simulink model "LIPMobsv"  (R2018b)
settings: Solver=VariableStepAuto  StartTime=0.0  StopTime=10.0  RelTol=1e-3
values from neighbouring files (symbols this model uses):
  arm_radius = leg_radius    (= 0.01)    [Nao_paramter.m]
  foot_height = 0.02    [Nao_paramter.m]
  foot_length = 0.1    [Nao_paramter.m]
  foot_mass = 0.17184    [Nao_paramter.m]
  foot_width = 0.05    [Nao_paramter.m]
  ground_height = 0.0025    [Nao_paramter.m]
  ground_length = 5    [Nao_paramter.m]
  ground_width = 2    [Nao_paramter.m]
  hand_mass = 0.18533    [Nao_paramter.m]
  head_mass = 0.60533    [Nao_paramter.m]
  hip_mass = 0.14053    [Nao_paramter.m]
  hip_off_Y = 0.05    [Nao_paramter.m]
  hip_off_Z = 0.085    [Nao_paramter.m]
  leg_radius = 0.01    [Nao_paramter.m]
  lowerarm_length = 0.05595    [Nao_paramter.m]
  lowerarm_mass = 0.07761    [Nao_paramter.m]
  neck_length = 0.03    [Nao_paramter.m]
  neck_mass = 0.07842    [Nao_paramter.m]
  neck_off_Z = 0.1265    [Nao_paramter.m]
  shoulder_mass = 0.09304    [Nao_paramter.m]
  thigh_mass = 0.38968    [Nao_paramter.m]
  tibia_mass = 0.30142    [Nao_paramter.m]
  torso_height = foot_height + tibia_length + thigh_length + 0.5*hip_off_Z    (= 0.2654)    [Nao_paramter.m]
  torso_mass = 1.0496    [Nao_paramter.m]
  upperarm_length = 0.105    [Nao_paramter.m]
  upperarm_mass = 0.15777    [Nao_paramter.m]
undefined symbols (not defined in the file or in its folder): sigbuilder_block, X, Y, Z
libraries: sm_lib x166, nesl_utility x34, Contact_Forces_Lib x20
(part 6 of 6)

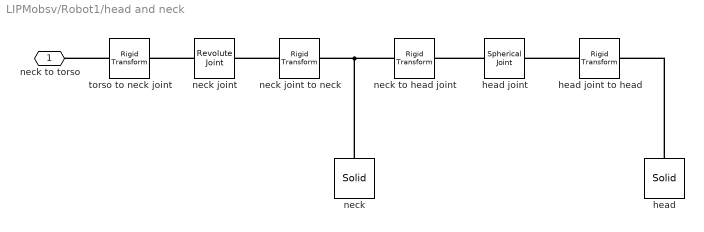
== system LIPMobsv/Robot1/head and neck ==
  head : sm_lib/Body Elements/Solid  InertiaType=CalculateFromGeometry  Mass=head_mass  MassUnits=kg  CenterOfMass=[0 0 0]  CenterOfMassUnits=m  MomentsOfInertia=[1 1 1]  MomentsOfInertiaUnits=kg*m^2  ProductsOfInertia=[1 1 1]  ProductsOfInertiaUnits=kg*m^2  BasedOnType=Mass  Density=1000  DensityUnits=kg/m^3  DoExposeReferenceFrame=on  SerializedFrames=<Frames/>  GraphicType=FromGeometry  MarkerShape=Sphere  MarkerSize=10  GraphicVisPropType=SimpleVisualProperties  GraphicDiffuseColor=[1.0 0.0 0.2]  GraphicSpecularColor=[0.5 0.5 0.5 1.0]  GraphicAmbientColor=[0.15 0.15 0.15 1.0]  GraphicEmissiveColor=[0.0 0.0 0.0 1.0]  GraphicShininess=75  GraphicOpacity=1.0  GeometryShape=Brick  RectangleSize=[1 1]  RectangleSizeUnits=m  BrickDimensions=[0.05 0.07 0.05]  BrickDimensionUnits=m  CylinderRadius=1  CylinderRadiusUnits=m  CylinderLength=1  CylinderLengthUnits=m  SphereRadius=1  SphereRadiusUnits=m  EllipsoidRadii=[1 1 1]  EllipsoidRadiiUnits=m  ExtrusionCrossSection=[1 1; -1 1; -1 -1; 1 -1]  ExtrusionCrossSectionUnits=m  ExtrusionLength=1  ExtrusionLengthUnits=m  PolygonNumSides=3  PolygonOuterRadius=1  PolygonOuterRadiusUnits=m  ExtGeomFileType=STEP  ExtGeomFileUnits=m  RevolutionCrossSection=[1 1; 1 -1; 2 -1; 2 1]  RevolutionCrossSectionUnits=m  RevolutionExtent=Full  RevolutionAngle=180  RevolutionAngleUnits=deg
  head joint : sm_lib/Joints/Spherical Joint  SenseConstraintForce=off  SenseConstraintForceX=off  SenseConstraintForceY=off  SenseConstraintForceZ=off  SenseConstraintTorque=off  SenseConstraintTorqueX=off  SenseConstraintTorqueY=off  SenseConstraintTorqueZ=off  SenseTotalForce=off  SenseTotalForceX=off  SenseTotalForceY=off  SenseTotalForceZ=off  SenseTotalTorque=off  SenseTotalTorqueX=off  SenseTotalTorqueY=off  SenseTotalTorqueZ=off  CompositeWrenchDir=FollowerOnBase  CompositeWrenchFrame=BaseFrame  DefPosRotationMethod=None  DefPosRotationAngleUnits=deg  DefPosRotationStandardAxis=+Z  DefPosRotationAngle=0.0  DefPosRotationArbitraryAxis=[0 0 1]  DefPosFollAlignAxisA=+X  DefPosBaseAlignAxisA=+Y  DefPosFollAlignAxisB=+Y  DefPosBaseAlignAxisB=+Z  DefPosRotationSequenceAxes=FollowerAxes  DefPosRotationSequence=XYX  DefPosRotationSequenceAngles=[0 0 0]  DefPosRotationSequenceAnglesUnits=deg  DefPosRotationMatrix=[1 0 0; 0 1 0; 0 0 1]  EqPosRotationMethod=None  EqPosRotationAngleUnits=deg  EqPosRotationStandardAxis=+Z  EqPosRotationAngle=0.0  EqPosRotationArbitraryAxis=[0 0 1]  EqPosFollAlignAxisA=+X  EqPosBaseAlignAxisA=+Y  EqPosFollAlignAxisB=+Y  EqPosBaseAlignAxisB=+Z  EqPosRotationSequenceAxes=FollowerAxes  EqPosRotationSequence=XYX  EqPosRotationSequenceAngles=[0 0 0]  EqPosRotationSequenceAnglesUnits=deg  EqPosRotationMatrix=[1 0 0; 0 1 0; 0 0 1]  SpringStiffness=0  SpringStiffnessUnits=N*m/deg  DampingCoefficient=0  DampingCoefficientUnits=N*m/(deg/s)  ActuateTorqueX=off  ActuateTorqueY=off  ActuateTorqueZ=off  ActuateTorque=off  TorqueActuationMode=NoTorque  MotionActuationMode=ComputedMotion  ActuationFrame=BaseFrame  SensePosition=off  SenseVelocityX=off  SenseVelocityY=off  SenseVelocityZ=off  SenseVelocity=off  SenseAccelerationX=off  SenseAccelerationY=off  SenseAccelerationZ=off  SenseAcceleration=off  SenseTorqueX=off  SenseTorqueY=off  SenseTorqueZ=off  SenseTorqueForce=off  SensingFrame=BaseFrame  PositionTargetRotationMethod=StandardAxis  PositionTargetRotationAngleUnits=deg  PositionTargetRotationStandardAxis=+Y  PositionTargetRotationAngle=5  PositionTargetRotationArbitraryAxis=[0 0 1]  PositionTargetFollAlignAxisA=+X  PositionTargetBaseAlignAxisA=+Y  PositionTargetFollAlignAxisB=+Y  PositionTargetBaseAlignAxisB=+Z  PositionTargetRotationSequenceAxes=FollowerAxes  PositionTargetRotationSequence=XYX  PositionTargetRotationSequenceAngles=[0 0 0]  PositionTargetRotationSequenceAnglesUnits=deg  PositionTargetRotationMatrix=[1 0 0; 0 1 0; 0 0 1]  PositionTargetSpecify=off  PositionTargetPriority=High  VelocityTargetValue=[0 0 0]  VelocityTargetValueUnits=deg/s  VelocityTargetSpecify=off  VelocityTargetPriority=High  VelocityTargetInFollowerFrame=on
  head joint to head : sm_lib/Frames and Transforms/Rigid Transform  TranslationMethod=StandardAxis  TranslationStandardOffset=0.025  TranslationLengthUnit=m  TranslationStandardAxis=+Z  TranslationCartesianOffset=[0 0 0]  TranslationROffset=0  TranslationROffsetUnits=m  TranslationZOffset=0  TranslationZOffsetUnits=m  TranslationThetaOffset=0  TranslationThetaOffsetUnits=deg  RotationMethod=None  RotationAngleUnits=deg  RotationStandardAxis=+Z  RotationAngle=0.0  RotationArbitraryAxis=[0 0 1]  FollAlignAxisA=+X  BaseAlignAxisA=+Y  FollAlignAxisB=+Y  BaseAlignAxisB=+Z  RotationSequenceAxes=FollowerAxes  RotationSequence=XYX  RotationSequenceAngles=[0 0 0]  RotationSequenceAnglesUnits=deg  RotationMatrix=[1 0 0; 0 1 0; 0 0 1]
  neck : sm_lib/Body Elements/Solid  InertiaType=CalculateFromGeometry  Mass=neck_mass  MassUnits=kg  CenterOfMass=[0 0 0]  CenterOfMassUnits=m  MomentsOfInertia=[1 1 1]  MomentsOfInertiaUnits=kg*m^2  ProductsOfInertia=[1 1 1]  ProductsOfInertiaUnits=kg*m^2  BasedOnType=Mass  Density=1000  DensityUnits=kg/m^3  DoExposeReferenceFrame=on  SerializedFrames=<Frames/>  GraphicType=FromGeometry  MarkerShape=Sphere  MarkerSize=10  GraphicVisPropType=SimpleVisualProperties  GraphicDiffuseColor=[0.5 0.5 0.5]  GraphicSpecularColor=[0.5 0.5 0.5 1.0]  GraphicAmbientColor=[0.15 0.15 0.15 1.0]  GraphicEmissiveColor=[0.0 0.0 0.0 1.0]  GraphicShininess=75  GraphicOpacity=1.0  GeometryShape=Cylinder  RectangleSize=[1 1]  RectangleSizeUnits=m  BrickDimensions=[1 1 1]  BrickDimensionUnits=m  CylinderRadius=neck_radius  CylinderRadiusUnits=m  CylinderLength=neck_length  CylinderLengthUnits=m  SphereRadius=1  SphereRadiusUnits=m  EllipsoidRadii=[1 1 1]  EllipsoidRadiiUnits=m  ExtrusionCrossSection=[1 1; -1 1; -1 -1; 1 -1]  ExtrusionCrossSectionUnits=m  ExtrusionLength=1  ExtrusionLengthUnits=m  PolygonNumSides=3  PolygonOuterRadius=1  PolygonOuterRadiusUnits=m  ExtGeomFileType=STEP  ExtGeomFileUnits=m  RevolutionCrossSection=[1 1; 1 -1; 2 -1; 2 1]  RevolutionCrossSectionUnits=m  RevolutionExtent=Full  RevolutionAngle=180  RevolutionAngleUnits=deg
  neck joint : sm_lib/Joints/Revolute Joint  SenseConstraintForce=off  SenseConstraintForceX=off  SenseConstraintForceY=off  SenseConstraintForceZ=off  SenseConstraintTorque=off  SenseConstraintTorqueX=off  SenseConstraintTorqueY=off  SenseConstraintTorqueZ=off  SenseTotalForce=off  SenseTotalForceX=off  SenseTotalForceY=off  SenseTotalForceZ=off  SenseTotalTorque=off  SenseTotalTorqueX=off  SenseTotalTorqueY=off  SenseTotalTorqueZ=off  CompositeWrenchDir=FollowerOnBase  CompositeWrenchFrame=BaseFrame  EquilibriumPosition=0  EquilibriumPositionUnits=deg  SpringStiffness=0  SpringStiffnessUnits=N*m/deg  DampingCoefficient=0  DampingCoefficientUnits=N*m/(deg/s)  TorqueActuationMode=NoTorque  MotionActuationMode=ComputedMotion  SensePosition=off  SenseVelocity=off  SenseAcceleration=off  SenseTorqueForce=off  PositionTargetSpecify=off  PositionTargetPriority=High  PositionTargetValue=0  PositionTargetValueUnits=deg  VelocityTargetSpecify=off  VelocityTargetPriority=High  VelocityTargetValue=0  VelocityTargetValueUnits=deg/s
  neck joint to neck : sm_lib/Frames and Transforms/Rigid Transform  TranslationMethod=None  TranslationStandardOffset=0  TranslationLengthUnit=m  TranslationStandardAxis=+Z  TranslationCartesianOffset=[0 0 0]  TranslationROffset=0  TranslationROffsetUnits=m  TranslationZOffset=0  TranslationZOffsetUnits=m  TranslationThetaOffset=0  TranslationThetaOffsetUnits=deg  RotationMethod=None  RotationAngleUnits=deg  RotationStandardAxis=+Z  RotationAngle=0.0  RotationArbitraryAxis=[0 0 1]  FollAlignAxisA=+X  BaseAlignAxisA=+Y  FollAlignAxisB=+Y  BaseAlignAxisB=+Z  RotationSequenceAxes=FollowerAxes  RotationSequence=XYX  RotationSequenceAngles=[0 0 0]  RotationSequenceAnglesUnits=deg  RotationMatrix=[1 0 0; 0 1 0; 0 0 1]
  neck to head joint : sm_lib/Frames and Transforms/Rigid Transform  TranslationMethod=StandardAxis  TranslationStandardOffset=neck_length/2  TranslationLengthUnit=m  TranslationStandardAxis=+Z  TranslationCartesianOffset=[0 0 0]  TranslationROffset=0  TranslationROffsetUnits=m  TranslationZOffset=0  TranslationZOffsetUnits=m  TranslationThetaOffset=0  TranslationThetaOffsetUnits=deg  RotationMethod=None  RotationAngleUnits=deg  RotationStandardAxis=+Z  RotationAngle=0.0  RotationArbitraryAxis=[0 0 1]  FollAlignAxisA=+X  BaseAlignAxisA=+Y  FollAlignAxisB=+Y  BaseAlignAxisB=+Z  RotationSequenceAxes=FollowerAxes  RotationSequence=XYX  RotationSequenceAngles=[0 0 0]  RotationSequenceAnglesUnits=deg  RotationMatrix=[1 0 0; 0 1 0; 0 0 1]
  torso to neck joint : sm_lib/Frames and Transforms/Rigid Transform  TranslationMethod=StandardAxis  TranslationStandardOffset=(hip_off_Z+neck_off_Z)/2  TranslationLengthUnit=m  TranslationStandardAxis=+Z  TranslationCartesianOffset=[0 0 0]  TranslationROffset=0  TranslationROffsetUnits=m  TranslationZOffset=0  TranslationZOffsetUnits=m  TranslationThetaOffset=0  TranslationThetaOffsetUnits=deg  RotationMethod=None  RotationAngleUnits=deg  RotationStandardAxis=+Z  RotationAngle=0.0  RotationArbitraryAxis=[0 0 1]  FollAlignAxisA=+X  BaseAlignAxisA=+Y  FollAlignAxisB=+Y  BaseAlignAxisB=+Z  RotationSequenceAxes=FollowerAxes  RotationSequence=XYX  RotationSequenceAngles=[0 0 0]  RotationSequenceAnglesUnits=deg  RotationMatrix=[1 0 0; 0 1 0; 0 0 1]
  neck to torso : PMIOPort  Side=Left
  connections:
  torso to neck joint/LConn1 -- neck to torso/RConn1
  neck joint/LConn1 -- torso to neck joint/RConn1
  neck joint to neck/LConn1 -- neck joint/RConn1
  neck/RConn1 -- neck to head joint/LConn1 -- neck joint to neck/RConn1
  head joint/LConn1 -- neck to head joint/RConn1
  head/RConn1 -- head joint to head/RConn1
  head joint to head/LConn1 -- head joint/RConn1

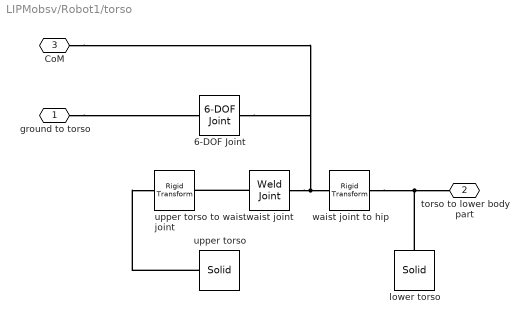
== system LIPMobsv/Robot1/torso ==
  " waist joint" : sm_lib/Joints/Weld Joint  SenseConstraintForce=off  SenseConstraintForceX=off  SenseConstraintForceY=off  SenseConstraintForceZ=off  SenseConstraintTorque=off  SenseConstraintTorqueX=off  SenseConstraintTorqueY=off  SenseConstraintTorqueZ=off  SenseTotalForce=off  SenseTotalForceX=off  SenseTotalForceY=off  SenseTotalForceZ=off  SenseTotalTorque=off  SenseTotalTorqueX=off  SenseTotalTorqueY=off  SenseTotalTorqueZ=off  CompositeWrenchDir=FollowerOnBase  CompositeWrenchFrame=BaseFrame
  6-DOF Joint : sm_lib/Joints/6-DOF Joint  SenseConstraintForce=off  SenseConstraintForceX=off  SenseConstraintForceY=off  SenseConstraintForceZ=off  SenseConstraintTorque=off  SenseConstraintTorqueX=off  SenseConstraintTorqueY=off  SenseConstraintTorqueZ=off  SenseTotalForce=off  SenseTotalForceX=off  SenseTotalForceY=off  SenseTotalForceZ=off  SenseTotalTorque=off  SenseTotalTorqueX=off  SenseTotalTorqueY=off  SenseTotalTorqueZ=off  CompositeWrenchDir=FollowerOnBase  CompositeWrenchFrame=BaseFrame  PxEquilibriumPosition=0  PxEquilibriumPositionUnits=m  PxSpringStiffness=1000  PxSpringStiffnessUnits=N/m  PxDampingCoefficient=800  PxDampingCoefficientUnits=N/(m/s)  PxTorqueActuationMode=NoTorque  PxMotionActuationMode=ComputedMotion  PxSensePosition=off  PxSenseVelocity=off  PxSenseAcceleration=off  PxSenseTorqueForce=off  PxPositionTargetSpecify=on  PxPositionTargetPriority=High  PxPositionTargetValue=0  PxPositionTargetValueUnits=m  PxVelocityTargetSpecify=off  PxVelocityTargetPriority=High  PxVelocityTargetValue=0  PxVelocityTargetValueUnits=m/s  PyEquilibriumPosition=0  PyEquilibriumPositionUnits=m  PySpringStiffness=1000  PySpringStiffnessUnits=N/m  PyDampingCoefficient=800  PyDampingCoefficientUnits=N/(m/s)  PyTorqueActuationMode=NoTorque  PyMotionActuationMode=ComputedMotion  PySensePosition=off  PySenseVelocity=off  PySenseAcceleration=off  PySenseTorqueForce=off  PyPositionTargetSpecify=on  PyPositionTargetPriority=High  PyPositionTargetValue=0  PyPositionTargetValueUnits=m  PyVelocityTargetSpecify=off  PyVelocityTargetPriority=High  PyVelocityTargetValue=0  PyVelocityTargetValueUnits=m/s  PzEquilibriumPosition=0  PzEquilibriumPositionUnits=m  PzSpringStiffness=1000  PzSpringStiffnessUnits=N/m  PzDampingCoefficient=800  PzDampingCoefficientUnits=N/(m/s)  PzTorqueActuationMode=NoTorque  PzMotionActuationMode=ComputedMotion  PzSensePosition=off  PzSenseVelocity=off  PzSenseAcceleration=off  PzSenseTorqueForce=off  PzPositionTargetSpecify=on  PzPositionTargetPriority=High  PzPositionTargetValue=torso_height+0.001  PzPositionTargetValueUnits=m  PzVelocityTargetSpecify=off  PzVelocityTargetPriority=High  PzVelocityTargetValue=0  PzVelocityTargetValueUnits=m/s  SphDefPosRotationMethod=None  SphDefPosRotationAngleUnits=deg  SphDefPosRotationStandardAxis=+Z  SphDefPosRotationAngle=0.0  SphDefPosRotationArbitraryAxis=[0 0 1]  SphDefPosFollAlignAxisA=+X  SphDefPosBaseAlignAxisA=+Y  SphDefPosFollAlignAxisB=+Y  SphDefPosBaseAlignAxisB=+Z  SphDefPosRotationSequenceAxes=FollowerAxes  SphDefPosRotationSequence=XYX  SphDefPosRotationSequenceAngles=[0 0 0]  SphDefPosRotationSequenceAnglesUnits=deg  SphDefPosRotationMatrix=[1 0 0; 0 1 0; 0 0 1]  SphEqPosRotationMethod=None  SphEqPosRotationAngleUnits=deg  SphEqPosRotationStandardAxis=+Z  SphEqPosRotationAngle=0.0  SphEqPosRotationArbitraryAxis=[0 0 1]  SphEqPosFollAlignAxisA=+X  SphEqPosBaseAlignAxisA=+Y  SphEqPosFollAlignAxisB=+Y  SphEqPosBaseAlignAxisB=+Z  SphEqPosRotationSequenceAxes=FollowerAxes  SphEqPosRotationSequence=XYX  SphEqPosRotationSequenceAngles=[0 0 0]  SphEqPosRotationSequenceAnglesUnits=deg  SphEqPosRotationMatrix=[1 0 0; 0 1 0; 0 0 1]  SphSpringStiffness=1000  SphSpringStiffnessUnits=N*m/deg  SphDampingCoefficient=1000  SphDampingCoefficientUnits=N*m/(rad/s)  SphActuateTorqueX=off  SphActuateTorqueY=off  SphActuateTorqueZ=off  SphActuateTorque=off  SphTorqueActuationMode=NoTorque  SphMotionActuationMode=ComputedMotion  SphActuationFrame=BaseFrame  SphSensePosition=off  SphSenseVelocityX=off  SphSenseVelocityY=off  SphSenseVelocityZ=off  SphSenseVelocity=off  SphSenseAccelerationX=off  SphSenseAccelerationY=off  SphSenseAccelerationZ=off  SphSenseAcceleration=off  SphSenseTorqueX=off  SphSenseTorqueY=off  SphSenseTorqueZ=off  SphSenseTorqueForce=off  SphSensingFrame=BaseFrame  SphPositionTargetRotationMethod=None  SphPositionTargetRotationAngleUnits=deg  SphPositionTargetRotationStandardAxis=+Z  SphPositionTargetRotationAngle=0.0  SphPositionTargetRotationArbitraryAxis=[0 0 1]  SphPositionTargetFollAlignAxisA=+X  SphPositionTargetBaseAlignAxisA=+Y  SphPositionTargetFollAlignAxisB=+Y  SphPositionTargetBaseAlignAxisB=+Z  SphPositionTargetRotationSequenceAxes=FollowerAxes  SphPositionTargetRotationSequence=XYX  SphPositionTargetRotationSequenceAngles=[0 0 0]  SphPositionTargetRotationSequenceAnglesUnits=deg  SphPositionTargetRotationMatrix=eye(3)  SphPositionTargetSpecify=off  SphPositionTargetPriority=High  SphVelocityTargetValue=[0 0 0]  SphVelocityTargetValueUnits=deg/s  SphVelocityTargetSpecify=off  SphVelocityTargetPriority=High  SphVelocityTargetInFollowerFrame=on
  lower torso : sm_lib/Body Elements/Solid  InertiaType=CalculateFromGeometry  Mass=hip_mass  MassUnits=kg  CenterOfMass=[0 0 0]  CenterOfMassUnits=m  MomentsOfInertia=[1 1 1]  MomentsOfInertiaUnits=kg*m^2  ProductsOfInertia=[1 1 1]  ProductsOfInertiaUnits=kg*m^2  BasedOnType=Mass  Density=1000  DensityUnits=kg/m^3  DoExposeReferenceFrame=on  SerializedFrames=<Frames/>  GraphicType=FromGeometry  MarkerShape=Sphere  MarkerSize=10  GraphicVisPropType=SimpleVisualProperties  GraphicDiffuseColor=[0.6 0.6 0.6]  GraphicSpecularColor=[0.5 0.5 0.5 1.0]  GraphicAmbientColor=[0.15 0.15 0.15 1.0]  GraphicEmissiveColor=[0.0 0.0 0.0 1.0]  GraphicShininess=75  GraphicOpacity=1.0  GeometryShape=Brick  RectangleSize=[1 1]  RectangleSizeUnits=m  BrickDimensions=[0.5*foot_length 2*hip_off_Y hip_off_Z]  BrickDimensionUnits=m  CylinderRadius=1  CylinderRadiusUnits=m  CylinderLength=1  CylinderLengthUnits=m  SphereRadius=1  SphereRadiusUnits=m  EllipsoidRadii=[1 1 1]  EllipsoidRadiiUnits=m  ExtrusionCrossSection=[1 1; -1 1; -1 -1; 1 -1]  ExtrusionCrossSectionUnits=m  ExtrusionLength=1  ExtrusionLengthUnits=m  PolygonNumSides=3  PolygonOuterRadius=1  PolygonOuterRadiusUnits=m  ExtGeomFileType=STEP  ExtGeomFileUnits=m  RevolutionCrossSection=[1 1; 1 -1; 2 -1; 2 1]  RevolutionCrossSectionUnits=m  RevolutionExtent=Full  RevolutionAngle=180  RevolutionAngleUnits=deg
  upper torso : sm_lib/Body Elements/Solid  InertiaType=Custom  Mass=torso_mass  MassUnits=kg  CenterOfMass=[-0.00413 0 0.5*neck_off_Z]  CenterOfMassUnits=m  MomentsOfInertia=torso_inertia_m  MomentsOfInertiaUnits=kg*m^2  ProductsOfInertia=torso_inertia_p  ProductsOfInertiaUnits=kg*m^2  BasedOnType=Mass  Density=1000  DensityUnits=kg/m^3  DoExposeReferenceFrame=on  SerializedFrames=<Frames/>  GraphicType=FromGeometry  MarkerShape=Sphere  MarkerSize=10  GraphicVisPropType=SimpleVisualProperties  GraphicDiffuseColor=[0.5 0.5 0.5]  GraphicSpecularColor=[0.5 0.5 0.5 1.0]  GraphicAmbientColor=[0.15 0.15 0.15 1.0]  GraphicEmissiveColor=[0.0 0.0 0.0 1.0]  GraphicShininess=75  GraphicOpacity=1.0  GeometryShape=Brick  RectangleSize=[1 1]  RectangleSizeUnits=m  BrickDimensions=[2*hip_off_Y 2.5*foot_width neck_off_Z]  BrickDimensionUnits=m  CylinderRadius=1  CylinderRadiusUnits=m  CylinderLength=1  CylinderLengthUnits=m  SphereRadius=1  SphereRadiusUnits=m  EllipsoidRadii=[1 1 1]  EllipsoidRadiiUnits=m  ExtrusionCrossSection=[1 1; -1 1; -1 -1; 1 -1]  ExtrusionCrossSectionUnits=m  ExtrusionLength=1  ExtrusionLengthUnits=m  PolygonNumSides=3  PolygonOuterRadius=1  PolygonOuterRadiusUnits=m  ExtGeomFileType=STEP  ExtGeomFileUnits=m  RevolutionCrossSection=[1 1; 1 -1; 2 -1; 2 1]  RevolutionCrossSectionUnits=m  RevolutionExtent=Full  RevolutionAngle=180  RevolutionAngleUnits=deg
  upper torso to waist joint : sm_lib/Frames and Transforms/Rigid Transform  TranslationMethod=StandardAxis  TranslationStandardOffset=0.5*neck_off_Z  TranslationLengthUnit=m  TranslationStandardAxis=-Z  TranslationCartesianOffset=[0 0 0]  TranslationROffset=0  TranslationROffsetUnits=m  TranslationZOffset=0  TranslationZOffsetUnits=m  TranslationThetaOffset=0  TranslationThetaOffsetUnits=deg  RotationMethod=None  RotationAngleUnits=deg  RotationStandardAxis=+Z  RotationAngle=0.0  RotationArbitraryAxis=[0 0 1]  FollAlignAxisA=+X  BaseAlignAxisA=+Y  FollAlignAxisB=+Y  BaseAlignAxisB=+Z  RotationSequenceAxes=FollowerAxes  RotationSequence=XYX  RotationSequenceAngles=[0 0 0]  RotationSequenceAnglesUnits=deg  RotationMatrix=[1 0 0; 0 1 0; 0 0 1]
  waist joint to hip : sm_lib/Frames and Transforms/Rigid Transform  TranslationMethod=StandardAxis  TranslationStandardOffset=0.5*hip_off_Z  TranslationLengthUnit=m  TranslationStandardAxis=-Z  TranslationCartesianOffset=[0 0 0]  TranslationROffset=0  TranslationROffsetUnits=m  TranslationZOffset=0  TranslationZOffsetUnits=m  TranslationThetaOffset=0  TranslationThetaOffsetUnits=deg  RotationMethod=None  RotationAngleUnits=deg  RotationStandardAxis=+Z  RotationAngle=0.0  RotationArbitraryAxis=[0 0 1]  FollAlignAxisA=+X  BaseAlignAxisA=+Y  FollAlignAxisB=+Y  BaseAlignAxisB=+Z  RotationSequenceAxes=FollowerAxes  RotationSequence=XYX  RotationSequenceAngles=[0 0 0]  RotationSequenceAnglesUnits=deg  RotationMatrix=[1 0 0; 0 1 0; 0 0 1]
  ground to torso : PMIOPort  Side=Left
  torso to lower body part : PMIOPort  Port=2  Side=Right
  CoM : PMIOPort  Port=3  Side=Left
  connections:
  upper torso/RConn1 -- upper torso to waist joint/LConn1
  " waist joint"/RConn1 -- 6-DOF Joint/RConn1 -- CoM/RConn1 -- waist joint to hip/LConn1
  waist joint to hip/RConn1 -- lower torso/RConn1 -- torso to lower body part/RConn1
  " waist joint"/LConn1 -- upper torso to waist joint/RConn1
  ground to torso/RConn1 -- 6-DOF Joint/LConn1

== stateflow chart LIPMobsv/motion planning1 ==
  state stepPlanning
    entry:
    sStr = 0.03 ;       % forward step size
    sSi = 0.05;        % sideward step size
    H = 0.01;            % foot lifting height
    CoMY = 0.006;
    CoMX = sStr;
    sD = stepDurationCal(CoMY);
    state motionGenBeg
      entry:
      [hRor,hRol,hPir,hPil,hYar,hYal,kBer,kBel,aRor,aRol,aPir,aPil]=motionBeg(sD/2,sStr,sSi,H,CoMX,CoMY);
      state outBeg
        entry:
        j = j+1;
        hipRollR = hRor(j);
        hipRollL = hRol(j);
        hipPitchR = hPir(j);
        hipPitchL = hPil(j);
        hipYawR = hYar(j);
        hipYawL = hYal(j);
        kneeBendR = kBer(j);
        kneeBendL = kBel(j);
        ankleRollR = aRor(j);
        ankleRollL = aRol(j);
        anklePitchR = aPir(j);
        anklePitchL = aPil(j);
      (default) -> outBeg : {j = 0;}
      outBeg -> outBeg : after(sD/200,sec)
    state motionGenR
      entry:
      [hRor,hRol,hPir,hPil,hYar,hYal,kBer,kBel,aRor,aRol,aPir,aPil]=motionR(sD,sStr,sSi,H,CoMX,CoMY);
      state outR
        entry:
        j = j+1;
        hipRollR = hRor(j);
        hipRollL = hRol(j);
        hipPitchR = hPir(j);
        hipPitchL = hPil(j);
        hipYawR = hYar(j);
        hipYawL = hYal(j);
        kneeBendR = kBer(j);
        kneeBendL = kBel(j);
        ankleRollR = aRor(j);
        ankleRollL = aRol(j);
        anklePitchR = aPir(j);
        anklePitchL = aPil(j);
      (default) -> outR : {j = 0;}
      outR -> outR : after(sD/100,sec)
    state motionGenL
      entry:
      [hRor,hRol,hPir,hPil,hYar,hYal,kBer,kBel,aRor,aRol,aPir,aPil]=motionL(sD ,sStr,sSi,H,CoMX,CoMY);
      state outL
        entry:
        j = j+1;
        hipRollR = hRor(j);
        hipRollL = hRol(j);
        hipPitchR = hPir(j);
        hipPitchL = hPil(j);
        hipYawR = hYar(j);
        hipYawL = hYal(j);
        kneeBendR = kBer(j);
        kneeBendL = kBel(j);
        ankleRollR = aRor(j);
        ankleRollL = aRol(j);
        anklePitchR = aPir(j);
        anklePitchL = aPil(j);
      (default) -> outL : {j = 0;}
      outL -> outL : after(sD/100,sec)
    (default) -> motionGenBeg
    motionGenBeg -> motionGenL : after(sD/2,sec)
    motionGenL -> motionGenR : [j > 99]
    motionGenR -> motionGenL : [j > 99]
  (default) -> stepPlanning
  data: hRr function_output; hRl function_output; hPr function_output; hPl function_output; hYr function_output; hYl function_output; kBr function_output; kBl function_output; aRr function_output; aRl function_output; aPr function_output; aPl function_output; stepDuration function_input; stepStr function_input; stepSide function_input; liftH function_input; comx function_input; comy function_input; comy function_input; stepDuration function_output; hRr function_output; hRl function_output; hPr function_output; hPl function_output; hYr function_output; hYl function_output; kBr function_output; kBl function_output; aRr function_output; aRl function_output; aPr function_output; aPl function_output; stepDuration function_input; stepStr function_input; stepSide function_input; liftH function_input; comx function_input; comy function_input; hRr function_output; hRl function_output; hPr function_output; hPl function_output; hYr function_output; hYl function_output; kBr function_output; kBl function_output; aRr function_output; aRl function_output; aPr function_output; aPl function_output; stepDuration function_input; stepStr function_input; stepSide function_input; liftH function_input; comx function_input; comy function_input; hipRollL output; hipRollR output; hipPitchL output; hipPitchR output; hipYawL output; hipYawR output; kneeBendL output; kneeBendR output; k local; ankleRollL output; ankleRollR output; anklePitchL output; anklePitchR output; aPil local; aPir local; aRol local; aRor local; hPil local; hPir local; hRol local; hRor local; hYal local; hYar local; kBel local; kBer local; H local; sD local; sSi local; sStr local; j local; CoMOffy local; CoMX local; CoMY local
  function [hRr,hRl,hPr,hPl,hYr,hYl,kBr,kBl,aRr,aRl,aPr,aPl] = motionBeg(stepDuration,stepStr,...:
    | function [hRr,hRl,hPr,hPl,hYr,hYl,kBr,kBl,aRr,aRl,aPr,aPl] = motionBeg(stepDuration,stepStr,...
    |     stepSide,liftH,comx,comy)
    | CoMOffx = comx;  
    | CoMOffy = comy;
    | t = linspace(0,stepDuration,100);
    | 
    | L = 0.2029;
    | tt = stepDuration*[0 0.1 0.2 0.3 0.4 0.5 0.6 0.7 0.8 0.9 1];
    | % hip roll
    | hR1 = pi/2-acos(CoMOffy*sin(pi/stepDuration*tt(:,1))/L);
    | hR2 = pi/2-acos(CoMOffy*sin(pi/stepDuration*tt(:,4))/L);
    | hR3 = pi/2-acos(CoMOffy*sin(pi/stepDuration*tt(:,6))/L);
    | hR4 = pi/2-acos(CoMOffy*sin(pi/stepDuration*tt(:,8))/L);
    | hR5 = pi/2-acos(CoMOffy*sin(pi/stepDuration*tt(:,11))/L);
    | hRl = -pchip([tt(:,1),tt(:,4),tt(:,6),tt(:,8),tt(:,11)],[hR1,hR2,hR3,hR4,hR5],t);
    | hRr = hRl;
    | % right hip pitch
    | hPr1 = 0;%asin((stepStr/2)/(L*cos(hR1)));
    | hPr2 = 0.6*(-acos(((L*cos(hR3)-liftH)^2+0.1^2-0.1029^2)/(2*(L*cos(hR3)-liftH)*0.1)));
    | hPr3 = -acos(((L*cos(hR3)-liftH)^2+0.1^2-0.1029^2)/(2*(L*cos(hR3)-liftH)*0.1));
    | hPr4 = 1.2*hPr3;
    | hPr5 = -asin((stepStr/2)/(L*cos(hR5)));
    | hPr = pchip([tt(:,1),tt(:,4),tt(:,6),tt(:,8),tt(:,11)],[hPr1,hPr2,hPr3,hPr4,hPr5],t);
    | % left hip pitch
    | hPl1 = 0;
    | hPl2 = 0.2*asin((stepStr/2)/(L*cos(hR5)));
    | hPl3 = 0.5*asin((stepStr/2)/(L*cos(hR5)));
    | hPl4 = 0.8*asin((stepStr/2)/(L*cos(hR5)));
    | hPl5 = asin((stepStr/2)/(L*cos(hR5))); 
    | hPl = pchip([tt(:,1),tt(:,4),tt(:,6),tt(:,8),tt(:,11)],[hPl1,hPl2,hPl3,hPl4,hPl5],t);
    | % right hip yaw
    | hYr = pchip([tt(:,1),tt(:,4),tt(:,6),tt(:,8),tt(:,11)],[0 0 0 0 0],t);
    | % left hip yaw
    | hYl = pchip([tt(:,1),tt(:,4),tt(:,6),tt(:,8),tt(:,11)],[0 0 0 0 0],t);
    | % right knee bend
    | kBr1 = 0;
    | kBr2 = 0.6*(-pi+acos((+0.1^2+0.1029^2-(L*cos(hR3)-liftH)^2)/(2*0.1029*0.1)));
    | kBr3 = -pi+acos((+0.1^2+0.1029^2-(L*cos(hR3)-liftH)^2)/(2*0.1029*0.1));
    | kBr4 = 0.6*(-pi+acos((+0.1^2+0.1029^2-(L*cos(hR3)-liftH)^2)/(2*0.1029*0.1)));
    | kBr5 = 0;
    | kBr = pchip([tt(:,1),tt(:,4),tt(:,6),tt(:,8),tt(:,11)],[kBr1,kBr2,kBr3,kBr4,kBr5],t);
    | % left knee bend
    | kBl = pchip([tt(:,1),tt(:,4),tt(:,6),tt(:,8),tt(:,11)],[0 0 0 -0.2 -0.2],t);
    | % right angle pitch 
    | aPr = -hPr+kBr;
    | % left ankle pitch
    | aPl = -hPl+kBl;
    | % right ankle roll
    | aRl = -hRl;
    | % left ankle roll
    | aRr = -hRr;
  function stepDuration = stepDurationCal(comy):
    | function stepDuration = stepDurationCal(comy)
    | 
    | ry = 0.05;
    | ry1 = 0.05;
    | sy = 0;
    | x0y = ry-comy;
    | x0y1 = ry1-comy;
    | te = 0.1;
    | k = sqrt(9.81/0.333);
    | tb1 = asinh(x0y*sinh(k*te)/x0y1)/k;
    | temp = x0y*cosh(k*te)+x0y1*cosh(k*tb1);
    | vte = k*x0y*sinh(k*te);
    | deltate = (ry1+sy+ry-temp)/(2*vte);
    | te = te+deltate;
    | count = 0;
    | while(abs(deltate) >= 0.0001)
    |     tb1 = asinh(x0y*sinh(k*te)/x0y1)/k;
    |     temp = x0y*cosh(k*te)+x0y1*cosh(k*tb1);
    |     vte = k*x0y*sinh(k*te);
    |     deltate = (ry1+sy+ry-temp)/(2*vte);
    |     te = te+deltate;
    |     count = count + 1;
    | end
    | tb1 = asinh(x0y*sinh(k*te)/x0y1)/k;
    | stepDuration = 2*te;
  function [hRr,hRl,hPr,hPl,hYr,hYl,kBr,kBl,aRr,aRl,aPr,aPl] = motionL(stepDuration,stepStr,...:
    |  function [hRr,hRl,hPr,hPl,hYr,hYl,kBr,kBl,aRr,aRl,aPr,aPl] = motionL(stepDuration,stepStr,...
    |     stepSide,liftH,comx,comy)
    | CoMOffx = comx;  
    | CoMOffy = -comy;
    | t = linspace(0,stepDuration/2,100);
    | 
    | L = 0.2029;
    | tt = stepDuration/2*[0 0.1 0.2 0.3 0.4 0.5 0.6 0.7 0.8 0.9 1];
    | % hip roll
    | hR1 = pi/2-acos(CoMOffy*sin(pi/stepDuration*tt(:,1))/L);
    | hR2 = pi/2-acos(CoMOffy*sin(pi/stepDuration*tt(:,4))/L);
    | hR3 = pi/2-acos(CoMOffy*sin(pi/stepDuration*tt(:,6))/L);
    | hR4 = pi/2-acos(CoMOffy*sin(pi/stepDuration*tt(:,8))/L);
    | hR5 = pi/2-acos(CoMOffy*sin(pi/stepDuration*tt(:,11))/L);
    | hRl = -pchip([tt(:,1),tt(:,4),tt(:,6),tt(:,8),tt(:,11)],[hR1,hR2,hR3,hR4,hR5],t);
    | hRr = hRl;
    | % left hip pitch
    | hPl1 = asin((stepStr/2)/(L*cos(hR1)));
    | hPl2 = 0.6*asin((stepStr/2)/(L*cos(hR1)));
    | hPl3 = -acos(((L*cos(hR3)-liftH)^2+0.1^2-0.1029^2)/(2*(L*cos(hR3)-liftH)*0.1));
    | hPl4 = 1.2*hPl3;
    | hPl5 = -asin((stepStr/2)/(L*cos(hR5)));
    | hPl = pchip([tt(:,1),tt(:,4),tt(:,6),tt(:,8),tt(:,11)],[hPl1,hPl2,hPl3,hPl4,hPl5],t);
    | % right hip pitch
    | hPr1 = -asin((stepStr/2)/(L*cos(hR1)));
    | hPr2 = 0.6*hPr1;
    | hPr3 = 0;
    | hPr4 = 0.6*asin((stepStr/2)/(L*cos(hR5))); 
    | hPr5 = asin((stepStr/2)/(L*cos(hR5)));
    | hPr = pchip([tt(:,1),tt(:,4),tt(:,6),tt(:,8),tt(:,11)],[hPr1,hPr2,hPr3,hPr4,hPr5],t);
    | % right hip yaw
    | hYr = pchip([tt(:,1),tt(:,4),tt(:,6),tt(:,8),tt(:,11)],[0 0 0 0 0],t);
    | % left hip yaw
    | hYl = pchip([tt(:,1),tt(:,4),tt(:,6),tt(:,8),tt(:,11)],[0 0 0 0 0],t);
    | % right knee bend
    | kBl1 = -0.2;
    | kBl2 = 0.6*kBl1;
    | kBl3 = -pi+acos((+0.1^2+0.1029^2-(L*cos(hR3)-liftH)^2)/(2*0.1029*0.1));
    | kBl4 = 0.6*(-pi+acos((+0.1^2+0.1029^2-(L*cos(hR3)-liftH)^2)/(2*0.1029*0.1)));
    | kBl5 = 0;
    | kBl = pchip([tt(:,1),tt(:,4),tt(:,6),tt(:,8),tt(:,11)],[kBl1,kBl2,kBl3,kBl4,kBl5],t);
    | % left knee bend
    | kBr = pchip([tt(:,1),tt(:,4),tt(:,6),tt(:,8),tt(:,11)],[0 0 0 -0.2 -0.2],t);
    | % right angle pitch 
    | aPr = -hPr+kBr;
    | % left ankle pitch
    | aPl = -hPl+kBl;
    | % right ankle roll
    | aRl = -hRl;
    | % left ankle roll
    | aRr = -hRr;
  function [hRr,hRl,hPr,hPl,hYr,hYl,kBr,kBl,aRr,aRl,aPr,aPl] = motionR(stepDuration,stepStr,...:
    | function [hRr,hRl,hPr,hPl,hYr,hYl,kBr,kBl,aRr,aRl,aPr,aPl] = motionR(stepDuration,stepStr,...
    |     stepSide,liftH,comx,comy)
    | CoMOffx = comx;  
    | CoMOffy = comy;
    | t = linspace(0,stepDuration,100);
    | 
    | L = 0.2029;
    | tt = stepDuration*[0 0.1 0.2 0.3 0.4 0.5 0.6 0.7 0.8 0.9 1];
    | % hip roll
    | hR1 = pi/2-acos(CoMOffy*sin(pi/stepDuration*tt(:,1))/L);
    | hR2 = pi/2-acos(CoMOffy*sin(pi/stepDuration*tt(:,4))/L);
    | hR3 = pi/2-acos(CoMOffy*sin(pi/stepDuration*tt(:,6))/L);
    | hR4 = pi/2-acos(CoMOffy*sin(pi/stepDuration*tt(:,8))/L);
    | hR5 = pi/2-acos(CoMOffy*sin(pi/stepDuration*tt(:,11))/L);
    | hRl = -pchip([tt(:,1),tt(:,4),tt(:,6),tt(:,8),tt(:,11)],[hR1,hR2,hR3,hR4,hR5],t);
    | hRr = hRl;
    | % right hip pitch
    | hPr1 = asin((stepStr/2)/(L*cos(hR1)));
    | hPr2 = 0.6*asin((stepStr/2)/(L*cos(hR1)));
    | hPr3 = -acos(((L*cos(hR3)-liftH)^2+0.1^2-0.1029^2)/(2*(L*cos(hR3)-liftH)*0.1));
    | hPr4 = 1.2*hPr3;
    | hPr5 = -asin((stepStr/2)/(L*cos(hR5)));
    | hPr = pchip([tt(:,1),tt(:,4),tt(:,6),tt(:,8),tt(:,11)],[hPr1,hPr2,hPr3,hPr4,hPr5],t);
    | % left hip pitch
    | hPl1 = -asin((stepStr/2)/(L*cos(hR1)));
    | hPl2 = 0.6*hPl1;
    | hPl3 = 0;
    | hPl4 = 0.6*asin((stepStr/2)/(L*cos(hR5)));
    | hPl5 = asin((stepStr/2)/(L*cos(hR5))); 
    | hPl = pchip([tt(:,1),tt(:,4),tt(:,6),tt(:,8),tt(:,11)],[hPl1,hPl2,hPl3,hPl4,hPl5],t);
    | % right hip yaw
    | hYr = pchip([tt(:,1),tt(:,4),tt(:,6),tt(:,8),tt(:,11)],[0 0 0 0 0],t);
    | % left hip yaw
    | hYl = pchip([tt(:,1),tt(:,4),tt(:,6),tt(:,8),tt(:,11)],[0 0 0 0 0],t);
    | % right knee bend
    | kBr1 = -0.2;
    | kBr2 = 0.6*kBr1;
    | kBr3 = -pi+acos((+0.1^2+0.1029^2-(L*cos(hR3)-liftH)^2)/(2*0.1029*0.1));
    | kBr4 = 0.6*(-pi+acos((+0.1^2+0.1029^2-(L*cos(hR3)-liftH)^2)/(2*0.1029*0.1)));
    | kBr5 = 0;
    | kBr = pchip([tt(:,1),tt(:,4),tt(:,6),tt(:,8),tt(:,11)],[kBr1,kBr2,kBr3,kBr4,kBr5],t);
    | % left knee bend
    | kBl = pchip([tt(:,1),tt(:,4),tt(:,6),tt(:,8),tt(:,11)],[0 0 0 -0.2 -0.2],t);
    | % right angle pitch 
    | aPr = -hPr+kBr;
    | % left ankle pitch
    | aPl = -hPl+kBl;
    | % right ankle roll
    | aRl = -hRl;
    | % left ankle roll
    | aRr = -hRr;

== stateflow chart LIPMobsv/motion planning ==
  state stepPlanning
    entry:
    sStr = 0.03;       % forward step size
    sSi = 0.1;        % sideward step size
    H = 0.01;            % foot lifting height
    CoMYOff = 0.02;
    sD = stepDurationCal(CoMYOff);
    state motionGenBeg
      entry:
      [hRor,hRol,hPir,hPil,hYar,hYal,kBer,kBel,aRor,aRol,aPir,aPil]=motionBeg(sD/2,sStr,sSi,H,CoMX,CoMY);
      state outBeg
        entry:
        j = j+1;
        hipRollR = hRor(j);
        hipRollL = hRol(j);
        hipPitchR = hPir(j);
        hipPitchL = hPil(j);
        hipYawR = hYar(j);
        hipYawL = hYal(j);
        kneeBendR = kBer(j);
        kneeBendL = kBel(j);
        ankleRollR = aRor(j);
        ankleRollL = aRol(j);
        anklePitchR = aPir(j);
        anklePitchL = aPil(j);
      (default) -> outBeg : {j = 0;}
      outBeg -> outBeg : after(sD/100,sec)
    state motionGenR
      entry:
      [hRor,hRol,hPir,hPil,hYar,hYal,kBer,kBel,aRor,aRol,aPir,aPil]=motionR(sD,sStr,sSi,H,CoMX,CoMY);
      state outR
        entry:
        j = j+1;
        hipRollR = hRor(j);
        hipRollL = hRol(j);
        hipPitchR = hPir(j);
        hipPitchL = hPil(j);
        hipYawR = hYar(j);
        hipYawL = hYal(j);
        kneeBendR = kBer(j);
        kneeBendL = kBel(j);
        ankleRollR = aRor(j);
        ankleRollL = aRol(j);
        anklePitchR = aPir(j);
        anklePitchL = aPil(j);
      (default) -> outR : {j = 0;}
      outR -> outR : after(sD/100,sec)
    state motionGenL
      entry:
      [hRor,hRol,hPir,hPil,hYar,hYal,kBer,kBel,aRor,aRol,aPir,aPil]=motionL(sD,sStr,sSi,H,CoMX,CoMY);
      state outL
        entry:
        j = j+1;
        hipRollR = hRor(j);
        hipRollL = hRol(j);
        hipPitchR = hPir(j);
        hipPitchL = hPil(j);
        hipYawR = hYar(j);
        hipYawL = hYal(j);
        kneeBendR = kBer(j);
        kneeBendL = kBel(j);
        ankleRollR = aRor(j);
        ankleRollL = aRol(j);
        anklePitchR = aPir(j);
        anklePitchL = aPil(j);
      (default) -> outL : {j = 0;}
      outL -> outL : after(sD/100,sec)
    (default) -> motionGenBeg
    motionGenBeg -> motionGenL : after(sD,sec)
    motionGenL -> motionGenR : [j > 99]
    motionGenR -> motionGenL : [j > 99]
  state Balancing
  (default) -> stepPlanning
  stepPlanning -> Balancing : [AccY > 2000]
  data: comyoff function_input; stepDuration function_output; stepDuration function_input; comx function_output; comy function_output; comyoff function_input; hRr function_output; hRl function_output; hPr function_output; hPl function_output; hYr function_output; hYl function_output; kBr function_output; kBl function_output; aRr function_output; aRl function_output; aPr function_output; aPl function_output; stepDuration function_input; stepStr function_input; stepSide function_input; liftH function_input; comx function_input; comy function_input; hRr function_output; hRl function_output; hPr function_output; hPl function_output; hYr function_output; hYl function_output; kBr function_output; kBl function_output; aRr function_output; aRl function_output; aPr function_output; aPl function_output; stepDuration function_input; stepStr function_input; stepSide function_input; liftH function_input; comx function_input; comy function_input; hRr function_output; hRl function_output; hPr function_output; hPl function_output; hYr function_output; hYl function_output; kBr function_output; kBl function_output; aRr function_output; aRl function_output; aPr function_output; aPl function_output; stepDuration function_input; stepStr function_input; stepSide function_input; liftH function_input; comx function_input; comy function_input; hipRollL output; hipRollR output; hipPitchL output; hipPitchR output; hipYawL output; hipYawR output; kneeBendL output; kneeBendR output; k local; ankleRollL output; ankleRollR output; anklePitchL output; anklePitchR output; aPil local; aPir local; aRol local; aRor local; hPil local; hPir local; hRol local; hRor local; hYal local; hYar local; kBel local; kBer local; H local; sD local; sSi local; sStr local; j local; CoMOffy local; CoMX local; CoMY local; AccY input; CoMYMeasured input; CoMYOff local
  function stepDuration = stepDurationCal(comyoff):
    | function stepDuration = stepDurationCal(comyoff)
    | 
    | ry = 0.05;
    | ry1 = 0.05;
    | sy = 0;
    | x0y = ry-comyoff;
    | x0y1 = ry1-comyoff;
    | te = 0.1;
    | k = sqrt(9.81/0.333);
    | tb1 = asinh(x0y*sinh(k*te)/x0y1)/k;
    | temp = x0y*cosh(k*te)+x0y1*cosh(k*tb1);
    | vte = k*x0y*sinh(k*te);
    | deltate = (ry1+sy+ry-temp)/(2*vte);
    | te = te+deltate;
    | count = 0;
    | while(abs(deltate) >= 0.0001)
    |     tb1 = asinh(x0y*sinh(k*te)/x0y1)/k;
    |     temp = x0y*cosh(k*te)+x0y1*cosh(k*tb1);
    |     vte = k*x0y*sinh(k*te);
    |     deltate = (ry1+sy+ry-temp)/(2*vte);
    |     te = te+deltate;
    |     count = count + 1;
    | end
    | tb1 = asinh(x0y*sinh(k*te)/x0y1)/k;
    | stepDuration = te;
  function [comx,comy] = CoMGen(stepDuration,comyoff):
    | function [comx,comy] = CoMGen(stepDuration,comyoff)
    | t = 0:0.01:stepDuration;
    | k = sqrt(9.81/0.333);
    | comy = (0.05-comyoff)*cosh(k*t);
  function [hRr,hRl,hPr,hPl,hYr,hYl,kBr,kBl,aRr,aRl,aPr,aPl] = motionBeg(stepDuration,stepStr,...:
    | function [hRr,hRl,hPr,hPl,hYr,hYl,kBr,kBl,aRr,aRl,aPr,aPl] = motionBeg(stepDuration,stepStr,...
    |     stepSide,liftH,comx,comy)
    | CoMOffx = comx;  
    | CoMOffy = comy;
    | t = linspace(0,stepDuration,100);
    | 
    | L = 0.2029;
    | tt = stepDuration*[0 0.1 0.2 0.3 0.4 0.5 0.6 0.7 0.8 0.9 1];
    | % hip roll
    | hR1 = pi/2-acos(CoMOffy*sin(pi/stepDuration*tt(:,1))/L);
    | hR2 = pi/2-acos(CoMOffy*sin(pi/stepDuration*tt(:,4))/L);
    | hR3 = pi/2-acos(CoMOffy*sin(pi/stepDuration*tt(:,6))/L);
    | hR4 = pi/2-acos(CoMOffy*sin(pi/stepDuration*tt(:,8))/L);
    | hR5 = pi/2-acos(CoMOffy*sin(pi/stepDuration*tt(:,11))/L);
    | 
    | hRl = -pchip([tt(:,1),tt(:,4),tt(:,6),tt(:,8),tt(:,11)],[hR1,hR2,hR3,hR4,hR5],t);
    | hRr = hRl;
    | % left hip pitch
    | hPr1 = 0;%asin(2*CoMOffx/(L*cos(hR1)));
    | hPr2 = 0;
    | hPr3 = -asin(stepStr*sin(pi/stepDuration*tt(:,4))/sqrt((L*cos(hR2)-liftH)^2+...
    |     (stepStr*sin(pi/stepDuration*tt(:,4)))^2))-acos((0.1^2+(L*cos(hR2)-liftH)^2+...
    |     (stepStr*sin(pi/stepDuration*tt(:,4)))^2-0.1029^2)/(2*0.1*sqrt((L*cos(hR2)-liftH)^2+...
    |     (stepStr*sin(pi/stepDuration*tt(:,4)))^2)));
    | % hPr3 = -acos(((L*cos(hR3))^2+L^2-stepStr^2)/(2*L*cos(hR3)*L));
    | hPr4 = -asin(CoMOffx/(L*cos(hR4)));%-acos(((L*cos(hR4))^2+L^2-(stepStr*sin(pi/stepDuration*tt(:,8)))^2)/...
    | %     (2*(L*cos(hR4))*L));
    | hPr5 = -asin(CoMOffx/(L*cos(hR5)));
    | hPr = pchip([tt(:,1),tt(:,4),tt(:,6),tt(:,8),tt(:,11)],[hPr1,hPr2,hPr3,hPr4,hPr5],t);
    | % right hip pitch
    | hPl1 = 0;
    | hPl2 = atan(CoMOffx*sin(pi/stepDuration*tt(:,4))/(L*cos(hR2)));
    | hPl3 = atan(CoMOffx/(L*cos(hR3)));
    | hPl4 = atan(CoMOffx*sin(pi/stepDuration*tt(:,8))/(L*cos(hR4)));
    | hPl5 = asin(CoMOffx/(L*cos(hR5)));    
    | hPl = pchip([tt(:,1),tt(:,4),tt(:,6),tt(:,8),tt(:,11)],[hPl1,hPl2,hPl3,hPl4,hPl5],t);
    | % right hip yaw
    | hYr = pchip([tt(:,1),tt(:,4),tt(:,6),tt(:,8),tt(:,11)],[0 0 0 0 0],t);
    | % left hip yaw
    | hYl = pchip([tt(:,1),tt(:,4),tt(:,6),tt(:,8),tt(:,11)],[0 0 0 0 0],t);
    | % right knee bend
    | kBr1 = 0;
    | kBr2 = -pi+acos((0.1^2+0.1029^2-(L*cos(hR2)-liftH)^2-...
    |     (stepStr*sin(pi/stepDuration*tt(:,4)))^2)/(2*0.1*0.1029));
    | kBr3 = 0;
    | kBr4 = 0;
    | kBr5 = 0;
    | kBr = pchip([tt(:,1),tt(:,4),tt(:,6),tt(:,8),tt(:,11)],[kBr1,kBr2,kBr3,kBr4,kBr5],t);
    | % left knee bend
    | kBl = pchip([tt(:,1),tt(:,4),tt(:,6),tt(:,8),tt(:,11)],[0 0 0 0 0],t);
    | % right angle pitch 
    | aPr = -hPr+kBr;
    | % left ankle pitch
    | aPl = -hPl+kBl;
    | % right ankle roll
    | aRl = -hRl;
    | % left ankle roll
    | aRr = -hRr;
  function [hRr,hRl,hPr,hPl,hYr,hYl,kBr,kBl,aRr,aRl,aPr,aPl] = motionL(stepDuration,stepStr,...:
    | function [hRr,hRl,hPr,hPl,hYr,hYl,kBr,kBl,aRr,aRl,aPr,aPl] = motionL(stepDuration,stepStr,...
    |     stepSide,liftH,comx,comy)
    | CoMOffx = comx;  
    | CoMOffy = -comy;
    | t = linspace(0,stepDuration,100);
    | 
    | L = 0.2029;
    | tt = stepDuration*[0 0.1 0.2 0.3 0.4 0.5 0.6 0.7 0.8 0.9 1];
    | % hip roll
    | hR1 = pi/2-acos(CoMOffy*sin(pi/stepDuration*tt(:,1))/L);
    | hR2 = pi/2-acos(CoMOffy*sin(pi/stepDuration*tt(:,4))/L);
    | hR3 = pi/2-acos(CoMOffy*sin(pi/stepDuration*tt(:,6))/L);
    | hR4 = pi/2-acos(CoMOffy*sin(pi/stepDuration*tt(:,8))/L);
    | hR5 = pi/2-acos(CoMOffy*sin(pi/stepDuration*tt(:,11))/L);
    | 
    | hRl = -pchip([tt(:,1),tt(:,4),tt(:,6),tt(:,8),tt(:,11)],[hR1,hR2,hR3,hR4,hR5],t);
    | hRr = hRl;
    | % left hip pitch
    | hPl1 = asin(CoMOffx/(L*cos(hR1)));
    | hPl2 = 0;
    | hPl3 = -asin(stepStr*sin(pi/stepDuration*tt(:,4))/sqrt((L*cos(hR2)-liftH)^2+...
    |     (stepStr*sin(pi/stepDuration*tt(:,4)))^2))-acos((0.1^2+(L*cos(hR2)-liftH)^2+...
    |     (stepStr*sin(pi/stepDuration*tt(:,4)))^2-0.1029^2)/(2*0.1*sqrt((L*cos(hR2)-liftH)^2+...
    |     (stepStr*sin(pi/stepDuration*tt(:,4)))^2)));
    | % hPl3 = -acos(((L*cos(hR3))^2+L^2-stepStr^2)/(2*L*cos(hR3)*L));
    | hPl4 = -asin(CoMOffx/(L*cos(hR4)));%-acos(((L*cos(hR4))^2+L^2-(stepStr*sin(pi/stepDuration*tt(:,8)))^2)/...
    | %     (2*(L*cos(hR4))*L));
    | hPl5 = -asin(CoMOffx/(L*cos(hR5)));
    | hPl = pchip([tt(:,1),tt(:,4),tt(:,6),tt(:,8),tt(:,11)],[hPl1,hPl2,hPl3,hPl4,hPl5],t);
    | % right hip pitch
    | hPr1 = -asin(CoMOffx/(L*cos(hR1)));
    | hPr2 = atan(CoMOffx*sin(pi/stepDuration*tt(:,4))/(L*cos(hR2)));
    | hPr3 = atan(CoMOffx/(L*cos(hR3)));
    | hPr4 = atan(CoMOffx*sin(pi/stepDuration*tt(:,8))/(L*cos(hR4)));
    | hPr5 = asin(CoMOffx/(L*cos(hR5)));
    | hPr = pchip([tt(:,1),tt(:,4),tt(:,6),tt(:,8),tt(:,11)],[hPr1,hPr2,hPr3,hPr4,hPr5],t);
    | % right hip yaw
    | hYr = pchip([tt(:,1),tt(:,4),tt(:,6),tt(:,8),tt(:,11)],[0 0 0 0 0],t);
    | % left hip yaw
    | hYl = pchip([tt(:,1),tt(:,4),tt(:,6),tt(:,8),tt(:,11)],[0 0 0 0 0],t);
    | % right knee bend
    | kBl1 = -0.2;
    | kBl2 = -pi+acos((0.1^2+0.1029^2-(L*cos(hR2)-liftH)^2-...
    |     (stepStr*sin(pi/stepDuration*tt(:,4)))^2)/(2*0.1*0.1029));
    | kBl3 = 0;
    | kBl4 = 0;
    | kBl5 = 0;
    | kBl = pchip([tt(:,1),tt(:,4),tt(:,6),tt(:,8),tt(:,11)],[kBl1,kBl2,kBl3,kBl4,kBl5],t);
    | % left knee bend
    | kBr = pchip([tt(:,1),tt(:,4),tt(:,6),tt(:,8),tt(:,11)],[0 0 0 -0.2 -0.2],t);
    | % right angle pitch 
    | aPr = -hPr+kBr;
    | % left ankle pitch
    | aPl = -hPl+kBl;
    | % right ankle roll
    | aRl = -hRl;
    | % left ankle roll
    | aRr = -hRr;
  function [hRr,hRl,hPr,hPl,hYr,hYl,kBr,kBl,aRr,aRl,aPr,aPl] = motionR(stepDuration,stepStr,...:
    | function [hRr,hRl,hPr,hPl,hYr,hYl,kBr,kBl,aRr,aRl,aPr,aPl] = motionR(stepDuration,stepStr,...
    |     stepSide,liftH,comx,comy)
    | CoMOffx = comx;  
    | CoMOffy = comy;
    | t = linspace(0,stepDuration,100);
    | 
    | L = 0.2029;
    | tt = stepDuration*[0 0.1 0.2 0.3 0.4 0.5 0.6 0.7 0.8 0.9 1];
    | % hip roll
    | hR1 = pi/2-acos(CoMOffy*sin(pi/stepDuration*tt(:,1))/L);
    | hR2 = pi/2-acos(CoMOffy*sin(pi/stepDuration*tt(:,4))/L);
    | hR3 = pi/2-acos(CoMOffy*sin(pi/stepDuration*tt(:,6))/L);
    | hR4 = pi/2-acos(CoMOffy*sin(pi/stepDuration*tt(:,8))/L);
    | hR5 = pi/2-acos(CoMOffy*sin(pi/stepDuration*tt(:,11))/L);
    | 
    | hRl = -pchip([tt(:,1),tt(:,4),tt(:,6),tt(:,8),tt(:,11)],[hR1,hR2,hR3,hR4,hR5],t);
    | hRr = hRl;
    | % left hip pitch
    | hPr1 = asin(CoMOffx/(L*cos(hR1)));
    | hPr2 = 0;
    | hPr3 = -asin(stepStr*sin(pi/stepDuration*tt(:,4))/sqrt((L*cos(hR2)-liftH)^2+...
    |     (stepStr*sin(pi/stepDuration*tt(:,4)))^2))-acos((0.1^2+(L*cos(hR2)-liftH)^2+...
    |     (stepStr*sin(pi/stepDuration*tt(:,4)))^2-0.1029^2)/(2*0.1*sqrt((L*cos(hR2)-liftH)^2+...
    |     (stepStr*sin(pi/stepDuration*tt(:,4)))^2)));
    | % hPr3 = -acos(((L*cos(hR3))^2+L^2-stepStr^2)/(2*L*cos(hR3)*L));
    | hPr4 = -asin(CoMOffx/(L*cos(hR4)));%-acos(((L*cos(hR4))^2+L^2-(stepStr*sin(pi/stepDuration*tt(:,8)))^2)/...
    | %     (2*(L*cos(hR4))*L));
    | hPr5 = -asin(CoMOffx/(L*cos(hR5)));
    | hPr = pchip([tt(:,1),tt(:,4),tt(:,6),tt(:,8),tt(:,11)],[hPr1,hPr2,hPr3,hPr4,hPr5],t);
    | % right hip pitch
    | hPl1 = -asin(CoMOffx/(L*cos(hR1)));
    | hPl2 = atan(CoMOffx*sin(pi/stepDuration*tt(:,4))/(L*cos(hR2)));
    | hPl3 = atan(CoMOffx/(L*cos(hR3)));
    | hPl4 = atan(CoMOffx*sin(pi/stepDuration*tt(:,8))/(L*cos(hR4)));
    | hPl5 = asin(CoMOffx/(L*cos(hR5)));    
    | hPl = pchip([tt(:,1),tt(:,4),tt(:,6),tt(:,8),tt(:,11)],[hPl1,hPl2,hPl3,hPl4,hPl5],t);
    | % right hip yaw
    | hYr = pchip([tt(:,1),tt(:,4),tt(:,6),tt(:,8),tt(:,11)],[0 0 0 0 0],t);
    | % left hip yaw
    | hYl = pchip([tt(:,1),tt(:,4),tt(:,6),tt(:,8),tt(:,11)],[0 0 0 0 0],t);
    | % right knee bend
    | kBr1 = -0.2;
    | kBr2 = -pi+acos((0.1^2+0.1029^2-(L*cos(hR2)-liftH)^2-...
    |     (stepStr*sin(pi/stepDuration*tt(:,4)))^2)/(2*0.1*0.1029));
    | kBr3 = 0;
    | kBr4 = 0;
    | kBr5 = 0;
    | kBr = pchip([tt(:,1),tt(:,4),tt(:,6),tt(:,8),tt(:,11)],[kBr1,kBr2,kBr3,kBr4,kBr5],t);
    | % left knee bend
    | kBl = pchip([tt(:,1),tt(:,4),tt(:,6),tt(:,8),tt(:,11)],[0 0 0 -0.2 -0.2],t);
    | % right angle pitch 
    | aPr = -hPr+kBr;
    | % left ankle pitch
    | aPl = -hPl+kBl;
    | % right ankle roll
    | aRl = -hRl;
    | % left ankle roll
    | aRr = -hRr;
